simulink model "Robot_holonome_cinematique"  (R2023a)
settings: Solver=VariableStepAuto  StartTime=0.0  StopTime=1000  RelTol=1e-3
libraries: slpidlib x4
settings Model: Creator=Matth_desm  LastModifiedBy=maxen
settings OptimizationCC: ReuseModelBlockBuffer=off

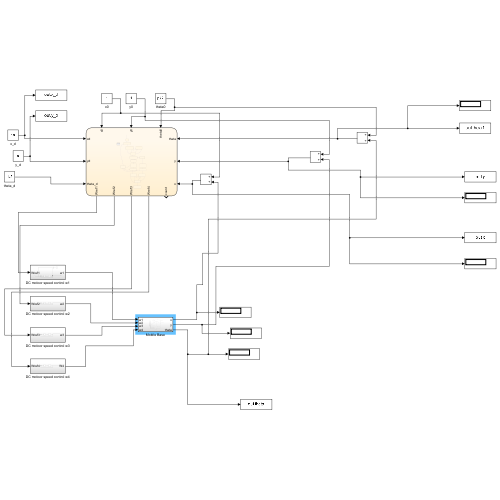
[thumbnail: Simulink's stored preview of the top-level diagram]
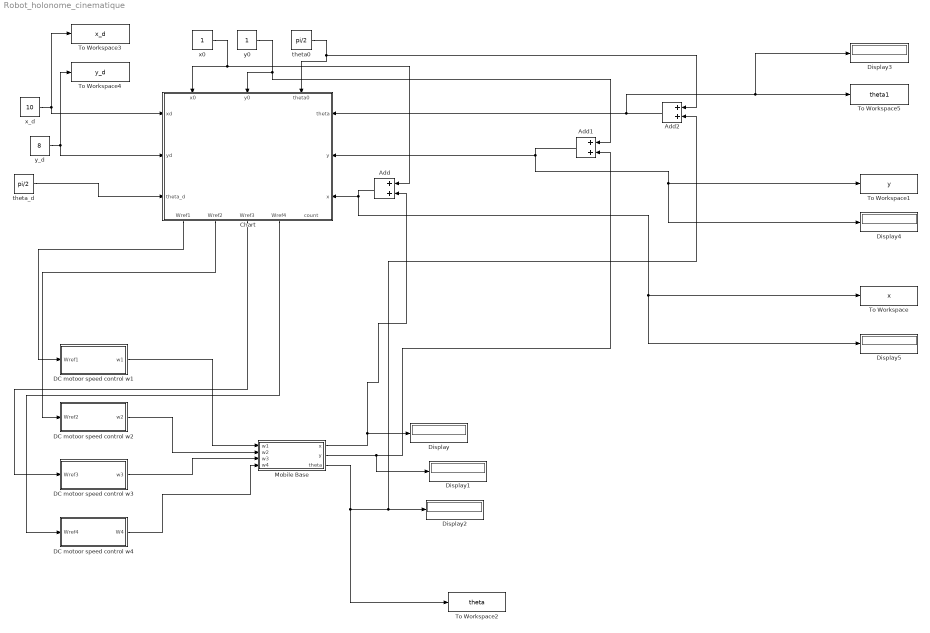
== system Robot_holonome_cinematique ==
  Add : Sum
  Add1 : Sum
  Add2 : Sum
  Chart : Stateflow chart  TreatAsAtomicUnit=on
      settings: PortSchema="{\"entries\":[{\"content\":{\"sides\":[{\"content\":{\"connectorIds\":[\"In5\",\"In6\",\"In3\"]},\"type\":\"ConnectorPlacement.EquallySpacedRectSide\",\"uuid\":\"9417ab48-c329-4538-ba36-cc7ccac6749b\"},{\"content\":{\"connectorIds\":[\"In7\",\"In8\",\"In9\"],\"side\":\"RIGHT\"},\"type\":\"ConnectorPlacement.EquallySpacedRectSide\",\"uuid\":\"8b0a8ded-c0e2-4ff2-a6eb-d9a6348e4391\"},{\"content\":{\"connectorIds\":[\"In1\",\"In2\",\"In4\"],\"side\":\"TOP\"},\"type\":\"ConnectorPlacement.EquallySpacedRectSide\",\"uuid\":\"84ebfe46-ef81-4416-a451-5548631499de\"},{\"content\":{\"connectorIds\":[\"Out1\",\"Out2\",\"Out3\",\"Out4\",\"Out5\"],\"side\":\"BOTTOM\"},\"type\":\"ConnectorPlacement.EquallySpacedRectSide\",\"uuid\":\"1f624b61-eefa-4aff-88e0-d3df134729c6\"}]},\"type\":\"ConnectorPlacement.EquallySpacedConnector\",\"uuid\":\"6488da51-1d08-4ec7-a718-29c3efed2e7e\"}],\"packageUris\":[\"http://schema.mathworks.com/mf0/Connector/R2020b\"],\"version\":\"1.0\"}"
  DC motoor speed control w1 : Subsystem
  DC motoor speed control w2 : Subsystem
  DC motoor speed control w3 : Subsystem
  DC motoor speed control w4 : Subsystem
  Display{,1..5} (6 alike) : Display
  Mobile Base : Subsystem
  To Workspace : ToWorkspace  VariableName=x  SampleTime=-1
      settings: Save2DSignal=2-D array (concatenate along first dimension)
  To Workspace1 : ToWorkspace  VariableName=y  SampleTime=-1
      settings: Save2DSignal=2-D array (concatenate along first dimension)
  To Workspace2 : ToWorkspace  VariableName=theta  SampleTime=-1
      settings: Save2DSignal=2-D array (concatenate along first dimension)
  To Workspace3 : ToWorkspace  VariableName=x_d  SampleTime=-1
      settings: Save2DSignal=2-D array (concatenate along first dimension)
  To Workspace4 : ToWorkspace  VariableName=y_d  SampleTime=-1
      settings: Save2DSignal=2-D array (concatenate along first dimension)
  To Workspace5 : ToWorkspace  VariableName=theta1  SampleTime=-1
      settings: Save2DSignal=2-D array (concatenate along first dimension)
  theta0 : Constant  Value=pi/2
  theta_d : Constant  Value=pi/2
  x0 : Constant
  x_d : Constant  Value=10
  y0 : Constant
  y_d : Constant  Value=8
  wires:
  DC motoor speed control w2/1(w2) -> Mobile Base/2(w2)
  DC motoor speed control w4/1(W4) -> Mobile Base/4(w4)
  Mobile Base/2(y) -> Add1/2, Display1/1
  DC motoor speed control w1/1(w1) -> Mobile Base/1(w1)
  Mobile Base/3(theta) -> To Workspace2/1, Add2/2, Display2/1
  Mobile Base/1(x) -> Add/2, Display/1
  DC motoor speed control w3/1(w3) -> Mobile Base/3(w3)
  theta0/1 -> Add2/1, Chart/4(theta0)
  x_d/1 -> To Workspace3/1, Chart/5(xd)
  theta_d/1 -> Chart/3(theta_d)
  y0/1 -> Add1/1, Chart/2(y0)
  x0/1 -> Add/1, Chart/1(x0)
  y_d/1 -> Chart/6(yd), To Workspace4/1
  Chart/1(Wref1) -> DC motoor speed control w1/1(Wref1)
  Chart/2(Wref2) -> DC motoor speed control w2/1(Wref2)
  Chart/3(Wref3) -> DC motoor speed control w3/1(Wref3)
  Chart/4(Wref4) -> DC motoor speed control w4/1(Wref4)
  Add1/1 -> Display4/1, To Workspace1/1, Chart/8(y)
  Add/1 -> Display5/1, To Workspace/1, Chart/9(x)
  Add2/1 -> Display3/1, To Workspace5/1, Chart/7(theta)

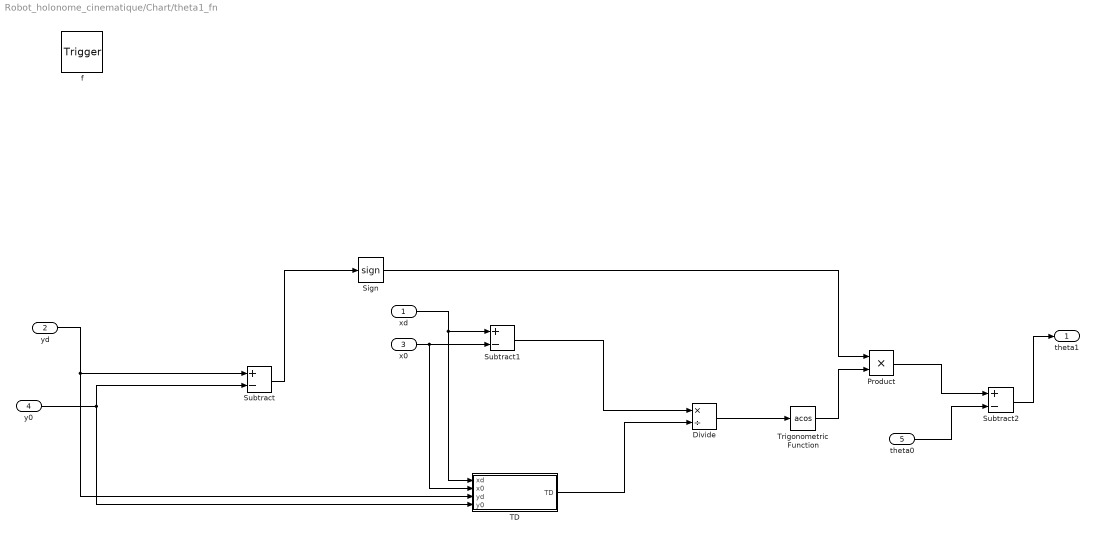
== system Robot_holonome_cinematique/Chart/theta1_fn ==
  xd : Inport  OutDataTypeStr=double  PortDimensions=1
  yd : Inport  Port=2  OutDataTypeStr=double  PortDimensions=1  LockScale=on
  x0 : Inport  Port=3  OutDataTypeStr=double  PortDimensions=1
  y0 : Inport  Port=4  OutDataTypeStr=double  PortDimensions=1
  theta0 : Inport  Port=5  OutDataTypeStr=double  PortDimensions=1
  f : TriggerPort  TriggerType=function-call  VariantControl=(inherit)
      settings: CopyFcn=Stateflow.SLINSF.SimulinkMan.removeBlockPreDeleteFcn  PreDeleteFcn=Stateflow.SLINSF.SimulinkMan.unsafePredeleteFcn
  Divide : Product  Inputs=*/
  Product : Product
  Sign : Signum
  Subtract : Sum  Inputs=+-
  Subtract1 : Sum  Inputs=+-
  Subtract2 : Sum  Inputs=+-
  TD : Subsystem
  Trigonometric Function : Trigonometry  Operator=acos
  theta1 : Outport  OutDataTypeStr=double
  wires:
  Trigonometric Function/1 -> Product/2
  TD/1(TD) -> Divide/2
  Sign/1 -> Product/1
  y0/1 -> TD/4(y0), Subtract/2
  Divide/1 -> Trigonometric Function/1
  Subtract1/1 -> Divide/1
  x0/1 -> TD/2(x0), Subtract1/2
  Subtract/1 -> Sign/1
  yd/1 -> TD/3(yd), Subtract/1
  xd/1 -> TD/1(xd), Subtract1/1
  Subtract2/1 -> theta1/1
  theta0/1 -> Subtract2/2
  Product/1 -> Subtract2/1

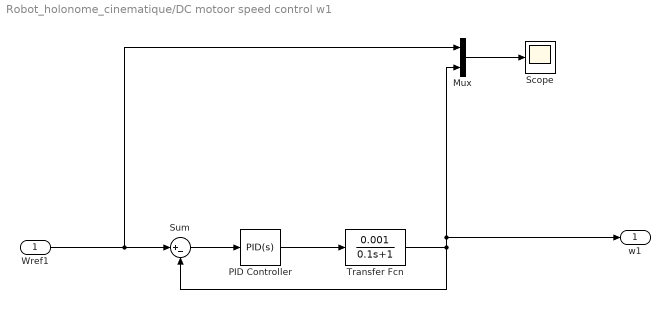
== system Robot_holonome_cinematique/DC motoor speed control w1 ==
  Wref1 : Inport
  Mux : Mux  Inputs=2
  PID Controller : slpidlib/PID Controller  Controller=PID  Form=Parallel  TimeDomain=Continuous-time  UseExternalTs=off  SampleTime=-1  IntegratorMethod=Forward Euler  FilterMethod=Forward Euler  ControllerParametersSource=internal  P=1337.5803137951  I=26735.5246643925  UseKiTs=off  D=-4.85758916096801  N=37.8094165182863  UseFilter=on  TunerSelectOption=Transfer Function Based (PID Tuner App)  InitialConditionSource=internal  InitialConditionForIntegrator=0  InitialConditionForFilter=0  DifferentiatorICPrevScaledInput=0  ExternalReset=none  TrackingMode=off  Kt=1  LimitOutput=off  SatLimitsSource=internal  UpperSaturationLimit=inf  LowerSaturationLimit=-inf  LinearizeAsGain=on  AntiWindupMode=none  Kb=1  LimitIntegrator=off  UpperIntegratorSaturationLimit=inf  LowerIntegratorSaturationLimit=-inf  POutMin=[]  POutMax=[]  IOutMin=[]  IOutMax=[]  DOutMin=[]  DOutMax=[]  NOutMin=[]  NOutMax=[]  SumOutMin=[]  SumOutMax=[]  SaturationOutMin=[]  SaturationOutMax=[]  PParamMin=[]  PParamMax=[]  IParamMin=[]  IParamMax=[]  DParamMin=[]  DParamMax=[]  NParamMin=[]  NParamMax=[]  KbParamMin=[]  KbParamMax=[]  KtParamMin=[]  KtParamMax=[]  KbOutMin=[]  KbOutMax=[]  KtOutMin=[]  KtOutMax=[]  IntegratorOutMin=[]  IntegratorOutMax=[]  FilterOutMin=[]  FilterOutMax=[]  SumI1OutMin=[]  SumI1OutMax=[]  SumI2OutMin=[]  SumI2OutMax=[]  SumI3OutMin=[]  SumI3OutMax=[]  SumI4OutMin=[]  SumI4OutMax=[]  SumDOutMin=[]  SumDOutMax=[]  DifferentiatorOutMin=[]  DifferentiatorOutMax=[]  FilterDiffOutCoefMin=[]  FilterDiffOutCoefMax=[]  ReciprocalOutMin=[]  ReciprocalOutMax=[]  SumDenOutMin=[]  SumDenOutMax=[]  SumNumOutMin=[]  SumNumOutMax=[]  DivideOutMin=[]  DivideOutMax=[]  UdiffTsProdOutMin=[]  UdiffTsProdOutMax=[]  NTsProdOutMin=[]  NTsProdOutMax=[]  UintegralTsProdOutMin=[]  UintegralTsProdOutMax=[]  UngainTsProdOutMin=[]  UngainTsProdOutMax=[]  ClampingZeroOutDataTypeStr=Inherit: Inherit via back propagation  ClampingZeroOutMin=[]  ClampingZeroOutMax=[]  FilterDenConstantOutDataTypeStr=Inherit: Inherit via back propagation  FilterDenConstantOutMin=[]  FilterDenConstantOutMax=[]  PCopyOutDataTypeStr=Inherit: Inherit via back propagation  PCopyOutMin=[]  PCopyOutMax=[]  NCopyOutDataTypeStr=Inherit: Inherit via back propagation  NCopyOutMin=[]  NCopyOutMax=[]  IntegratorContinuousStateAttributes=''  IntegratorStateMustResolveToSignalObject=off  IntegratorRTWStateStorageClass=Auto  FilterContinuousStateAttributes=''  FilterStateMustResolveToSignalObject=off  FilterRTWStateStorageClass=Auto  ParallelPVariant=InternalParameters  IdealPVariant=Disabled  IVariant=InternalParameters  DVariant=InternalParameters  IntegratorVariant=Continuous  SatVariant=Disabled  AWVariant=Passthrough  PCopyVariant=Disabled  TRVariant=Disabled  FdbkBlocksVariant=Forward  IdealPFdbkVariant=Disabled  SatFdbkVariant=Disabled  DerivativeFilterVariant=ContFilter  NVariant=InternalParameters  NCopyVariant=Disabled  FilterICVariant=InternalICsFilter  IntegratorICVariant=InternalICs  ExternalResetVariant=Disabled  TRSumVariant=Passthrough  SumFdbkVariant=Disabled  SumVariant=Sum_PID  TsampFilterVariant=InternalTs  TsampNgainVariant=Passthrough  TsampIntegralVariant=Disabled_SignalSpec  ExternalSaturationOutDataTypeStr=Inherit: Same as second input
  Scope : Scope
  Sum : Sum  Inputs=|+-
  Transfer Fcn : TransferFcn  Numerator=0.001  Denominator=[0.1 1]
  w1 : Outport
  wires:
  PID Controller/1 -> Transfer Fcn/1
  Transfer Fcn/1 -> Mux/2, w1/1, Sum/2
  Sum/1 -> PID Controller/1
  Wref1/1 -> Mux/1, Sum/1
  Mux/1 -> Scope/1

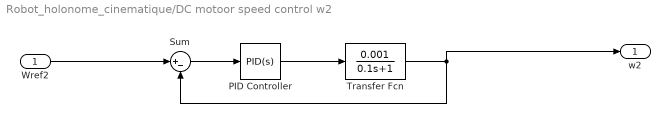
== system Robot_holonome_cinematique/DC motoor speed control w2 ==
  Wref2 : Inport
  PID Controller : slpidlib/PID Controller  Controller=PID  Form=Parallel  TimeDomain=Continuous-time  UseExternalTs=off  SampleTime=-1  IntegratorMethod=Forward Euler  FilterMethod=Forward Euler  ControllerParametersSource=internal  P=1337.5803137951  I=26735.5246643925  UseKiTs=off  D=-4.85758916096801  N=37.8094165182863  UseFilter=on  TunerSelectOption=Transfer Function Based (PID Tuner App)  InitialConditionSource=internal  InitialConditionForIntegrator=0  InitialConditionForFilter=0  DifferentiatorICPrevScaledInput=0  ExternalReset=none  TrackingMode=off  Kt=1  LimitOutput=off  SatLimitsSource=internal  UpperSaturationLimit=inf  LowerSaturationLimit=-inf  LinearizeAsGain=on  AntiWindupMode=none  Kb=1  LimitIntegrator=off  UpperIntegratorSaturationLimit=inf  LowerIntegratorSaturationLimit=-inf  POutMin=[]  POutMax=[]  IOutMin=[]  IOutMax=[]  DOutMin=[]  DOutMax=[]  NOutMin=[]  NOutMax=[]  SumOutMin=[]  SumOutMax=[]  SaturationOutMin=[]  SaturationOutMax=[]  PParamMin=[]  PParamMax=[]  IParamMin=[]  IParamMax=[]  DParamMin=[]  DParamMax=[]  NParamMin=[]  NParamMax=[]  KbParamMin=[]  KbParamMax=[]  KtParamMin=[]  KtParamMax=[]  KbOutMin=[]  KbOutMax=[]  KtOutMin=[]  KtOutMax=[]  IntegratorOutMin=[]  IntegratorOutMax=[]  FilterOutMin=[]  FilterOutMax=[]  SumI1OutMin=[]  SumI1OutMax=[]  SumI2OutMin=[]  SumI2OutMax=[]  SumI3OutMin=[]  SumI3OutMax=[]  SumI4OutMin=[]  SumI4OutMax=[]  SumDOutMin=[]  SumDOutMax=[]  DifferentiatorOutMin=[]  DifferentiatorOutMax=[]  FilterDiffOutCoefMin=[]  FilterDiffOutCoefMax=[]  ReciprocalOutMin=[]  ReciprocalOutMax=[]  SumDenOutMin=[]  SumDenOutMax=[]  SumNumOutMin=[]  SumNumOutMax=[]  DivideOutMin=[]  DivideOutMax=[]  UdiffTsProdOutMin=[]  UdiffTsProdOutMax=[]  NTsProdOutMin=[]  NTsProdOutMax=[]  UintegralTsProdOutMin=[]  UintegralTsProdOutMax=[]  UngainTsProdOutMin=[]  UngainTsProdOutMax=[]  ClampingZeroOutDataTypeStr=Inherit: Inherit via back propagation  ClampingZeroOutMin=[]  ClampingZeroOutMax=[]  FilterDenConstantOutDataTypeStr=Inherit: Inherit via back propagation  FilterDenConstantOutMin=[]  FilterDenConstantOutMax=[]  PCopyOutDataTypeStr=Inherit: Inherit via back propagation  PCopyOutMin=[]  PCopyOutMax=[]  NCopyOutDataTypeStr=Inherit: Inherit via back propagation  NCopyOutMin=[]  NCopyOutMax=[]  IntegratorContinuousStateAttributes=''  IntegratorStateMustResolveToSignalObject=off  IntegratorRTWStateStorageClass=Auto  FilterContinuousStateAttributes=''  FilterStateMustResolveToSignalObject=off  FilterRTWStateStorageClass=Auto  ParallelPVariant=InternalParameters  IdealPVariant=Disabled  IVariant=InternalParameters  DVariant=InternalParameters  IntegratorVariant=Continuous  SatVariant=Disabled  AWVariant=Passthrough  PCopyVariant=Disabled  TRVariant=Disabled  FdbkBlocksVariant=Forward  IdealPFdbkVariant=Disabled  SatFdbkVariant=Disabled  DerivativeFilterVariant=ContFilter  NVariant=InternalParameters  NCopyVariant=Disabled  FilterICVariant=InternalICsFilter  IntegratorICVariant=InternalICs  ExternalResetVariant=Disabled  TRSumVariant=Passthrough  SumFdbkVariant=Disabled  SumVariant=Sum_PID  TsampFilterVariant=InternalTs  TsampNgainVariant=Passthrough  TsampIntegralVariant=Disabled_SignalSpec  ExternalSaturationOutDataTypeStr=Inherit: Same as second input
  Sum : Sum  Inputs=|+-
  Transfer Fcn : TransferFcn  Numerator=0.001  Denominator=[0.1 1]
  w2 : Outport
  wires:
  PID Controller/1 -> Transfer Fcn/1
  Transfer Fcn/1 -> w2/1, Sum/2
  Sum/1 -> PID Controller/1
  Wref2/1 -> Sum/1

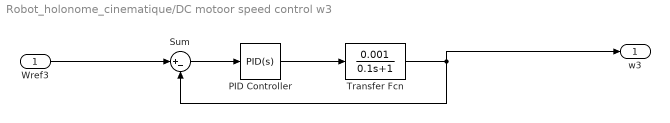
== system Robot_holonome_cinematique/DC motoor speed control w3 ==
  Wref3 : Inport
  PID Controller : slpidlib/PID Controller  Controller=PID  Form=Parallel  TimeDomain=Continuous-time  UseExternalTs=off  SampleTime=-1  IntegratorMethod=Forward Euler  FilterMethod=Forward Euler  ControllerParametersSource=internal  P=1337.5803137951  I=26735.5246643925  UseKiTs=off  D=-4.85758916096801  N=37.8094165182863  UseFilter=on  TunerSelectOption=Transfer Function Based (PID Tuner App)  InitialConditionSource=internal  InitialConditionForIntegrator=0  InitialConditionForFilter=0  DifferentiatorICPrevScaledInput=0  ExternalReset=none  TrackingMode=off  Kt=1  LimitOutput=off  SatLimitsSource=internal  UpperSaturationLimit=inf  LowerSaturationLimit=-inf  LinearizeAsGain=on  AntiWindupMode=none  Kb=1  LimitIntegrator=off  UpperIntegratorSaturationLimit=inf  LowerIntegratorSaturationLimit=-inf  POutMin=[]  POutMax=[]  IOutMin=[]  IOutMax=[]  DOutMin=[]  DOutMax=[]  NOutMin=[]  NOutMax=[]  SumOutMin=[]  SumOutMax=[]  SaturationOutMin=[]  SaturationOutMax=[]  PParamMin=[]  PParamMax=[]  IParamMin=[]  IParamMax=[]  DParamMin=[]  DParamMax=[]  NParamMin=[]  NParamMax=[]  KbParamMin=[]  KbParamMax=[]  KtParamMin=[]  KtParamMax=[]  KbOutMin=[]  KbOutMax=[]  KtOutMin=[]  KtOutMax=[]  IntegratorOutMin=[]  IntegratorOutMax=[]  FilterOutMin=[]  FilterOutMax=[]  SumI1OutMin=[]  SumI1OutMax=[]  SumI2OutMin=[]  SumI2OutMax=[]  SumI3OutMin=[]  SumI3OutMax=[]  SumI4OutMin=[]  SumI4OutMax=[]  SumDOutMin=[]  SumDOutMax=[]  DifferentiatorOutMin=[]  DifferentiatorOutMax=[]  FilterDiffOutCoefMin=[]  FilterDiffOutCoefMax=[]  ReciprocalOutMin=[]  ReciprocalOutMax=[]  SumDenOutMin=[]  SumDenOutMax=[]  SumNumOutMin=[]  SumNumOutMax=[]  DivideOutMin=[]  DivideOutMax=[]  UdiffTsProdOutMin=[]  UdiffTsProdOutMax=[]  NTsProdOutMin=[]  NTsProdOutMax=[]  UintegralTsProdOutMin=[]  UintegralTsProdOutMax=[]  UngainTsProdOutMin=[]  UngainTsProdOutMax=[]  ClampingZeroOutDataTypeStr=Inherit: Inherit via back propagation  ClampingZeroOutMin=[]  ClampingZeroOutMax=[]  FilterDenConstantOutDataTypeStr=Inherit: Inherit via back propagation  FilterDenConstantOutMin=[]  FilterDenConstantOutMax=[]  PCopyOutDataTypeStr=Inherit: Inherit via back propagation  PCopyOutMin=[]  PCopyOutMax=[]  NCopyOutDataTypeStr=Inherit: Inherit via back propagation  NCopyOutMin=[]  NCopyOutMax=[]  IntegratorContinuousStateAttributes=''  IntegratorStateMustResolveToSignalObject=off  IntegratorRTWStateStorageClass=Auto  FilterContinuousStateAttributes=''  FilterStateMustResolveToSignalObject=off  FilterRTWStateStorageClass=Auto  ParallelPVariant=InternalParameters  IdealPVariant=Disabled  IVariant=InternalParameters  DVariant=InternalParameters  IntegratorVariant=Continuous  SatVariant=Disabled  AWVariant=Passthrough  PCopyVariant=Disabled  TRVariant=Disabled  FdbkBlocksVariant=Forward  IdealPFdbkVariant=Disabled  SatFdbkVariant=Disabled  DerivativeFilterVariant=ContFilter  NVariant=InternalParameters  NCopyVariant=Disabled  FilterICVariant=InternalICsFilter  IntegratorICVariant=InternalICs  ExternalResetVariant=Disabled  TRSumVariant=Passthrough  SumFdbkVariant=Disabled  SumVariant=Sum_PID  TsampFilterVariant=InternalTs  TsampNgainVariant=Passthrough  TsampIntegralVariant=Disabled_SignalSpec  ExternalSaturationOutDataTypeStr=Inherit: Same as second input
  Sum : Sum  Inputs=|+-
  Transfer Fcn : TransferFcn  Numerator=0.001  Denominator=[0.1 1]
  w3 : Outport
  wires:
  PID Controller/1 -> Transfer Fcn/1
  Transfer Fcn/1 -> w3/1, Sum/2
  Sum/1 -> PID Controller/1
  Wref3/1 -> Sum/1

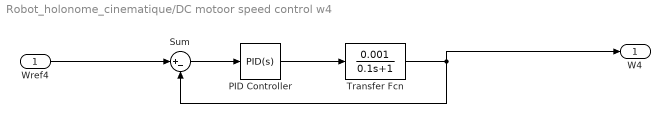
== system Robot_holonome_cinematique/DC motoor speed control w4 ==
  Wref4 : Inport
  PID Controller : slpidlib/PID Controller  Controller=PID  Form=Parallel  TimeDomain=Continuous-time  UseExternalTs=off  SampleTime=-1  IntegratorMethod=Forward Euler  FilterMethod=Forward Euler  ControllerParametersSource=internal  P=1337.5803137951  I=26735.5246643925  UseKiTs=off  D=-4.85758916096801  N=37.8094165182863  UseFilter=on  TunerSelectOption=Transfer Function Based (PID Tuner App)  InitialConditionSource=internal  InitialConditionForIntegrator=0  InitialConditionForFilter=0  DifferentiatorICPrevScaledInput=0  ExternalReset=none  TrackingMode=off  Kt=1  LimitOutput=off  SatLimitsSource=internal  UpperSaturationLimit=inf  LowerSaturationLimit=-inf  LinearizeAsGain=on  AntiWindupMode=none  Kb=1  LimitIntegrator=off  UpperIntegratorSaturationLimit=inf  LowerIntegratorSaturationLimit=-inf  POutMin=[]  POutMax=[]  IOutMin=[]  IOutMax=[]  DOutMin=[]  DOutMax=[]  NOutMin=[]  NOutMax=[]  SumOutMin=[]  SumOutMax=[]  SaturationOutMin=[]  SaturationOutMax=[]  PParamMin=[]  PParamMax=[]  IParamMin=[]  IParamMax=[]  DParamMin=[]  DParamMax=[]  NParamMin=[]  NParamMax=[]  KbParamMin=[]  KbParamMax=[]  KtParamMin=[]  KtParamMax=[]  KbOutMin=[]  KbOutMax=[]  KtOutMin=[]  KtOutMax=[]  IntegratorOutMin=[]  IntegratorOutMax=[]  FilterOutMin=[]  FilterOutMax=[]  SumI1OutMin=[]  SumI1OutMax=[]  SumI2OutMin=[]  SumI2OutMax=[]  SumI3OutMin=[]  SumI3OutMax=[]  SumI4OutMin=[]  SumI4OutMax=[]  SumDOutMin=[]  SumDOutMax=[]  DifferentiatorOutMin=[]  DifferentiatorOutMax=[]  FilterDiffOutCoefMin=[]  FilterDiffOutCoefMax=[]  ReciprocalOutMin=[]  ReciprocalOutMax=[]  SumDenOutMin=[]  SumDenOutMax=[]  SumNumOutMin=[]  SumNumOutMax=[]  DivideOutMin=[]  DivideOutMax=[]  UdiffTsProdOutMin=[]  UdiffTsProdOutMax=[]  NTsProdOutMin=[]  NTsProdOutMax=[]  UintegralTsProdOutMin=[]  UintegralTsProdOutMax=[]  UngainTsProdOutMin=[]  UngainTsProdOutMax=[]  ClampingZeroOutDataTypeStr=Inherit: Inherit via back propagation  ClampingZeroOutMin=[]  ClampingZeroOutMax=[]  FilterDenConstantOutDataTypeStr=Inherit: Inherit via back propagation  FilterDenConstantOutMin=[]  FilterDenConstantOutMax=[]  PCopyOutDataTypeStr=Inherit: Inherit via back propagation  PCopyOutMin=[]  PCopyOutMax=[]  NCopyOutDataTypeStr=Inherit: Inherit via back propagation  NCopyOutMin=[]  NCopyOutMax=[]  IntegratorContinuousStateAttributes=''  IntegratorStateMustResolveToSignalObject=off  IntegratorRTWStateStorageClass=Auto  FilterContinuousStateAttributes=''  FilterStateMustResolveToSignalObject=off  FilterRTWStateStorageClass=Auto  ParallelPVariant=InternalParameters  IdealPVariant=Disabled  IVariant=InternalParameters  DVariant=InternalParameters  IntegratorVariant=Continuous  SatVariant=Disabled  AWVariant=Passthrough  PCopyVariant=Disabled  TRVariant=Disabled  FdbkBlocksVariant=Forward  IdealPFdbkVariant=Disabled  SatFdbkVariant=Disabled  DerivativeFilterVariant=ContFilter  NVariant=InternalParameters  NCopyVariant=Disabled  FilterICVariant=InternalICsFilter  IntegratorICVariant=InternalICs  ExternalResetVariant=Disabled  TRSumVariant=Passthrough  SumFdbkVariant=Disabled  SumVariant=Sum_PID  TsampFilterVariant=InternalTs  TsampNgainVariant=Passthrough  TsampIntegralVariant=Disabled_SignalSpec  ExternalSaturationOutDataTypeStr=Inherit: Same as second input
  Sum : Sum  Inputs=|+-
  Transfer Fcn : TransferFcn  Numerator=0.001  Denominator=[0.1 1]
  W4 : Outport
  wires:
  PID Controller/1 -> Transfer Fcn/1
  Transfer Fcn/1 -> W4/1, Sum/2
  Sum/1 -> PID Controller/1
  Wref4/1 -> Sum/1

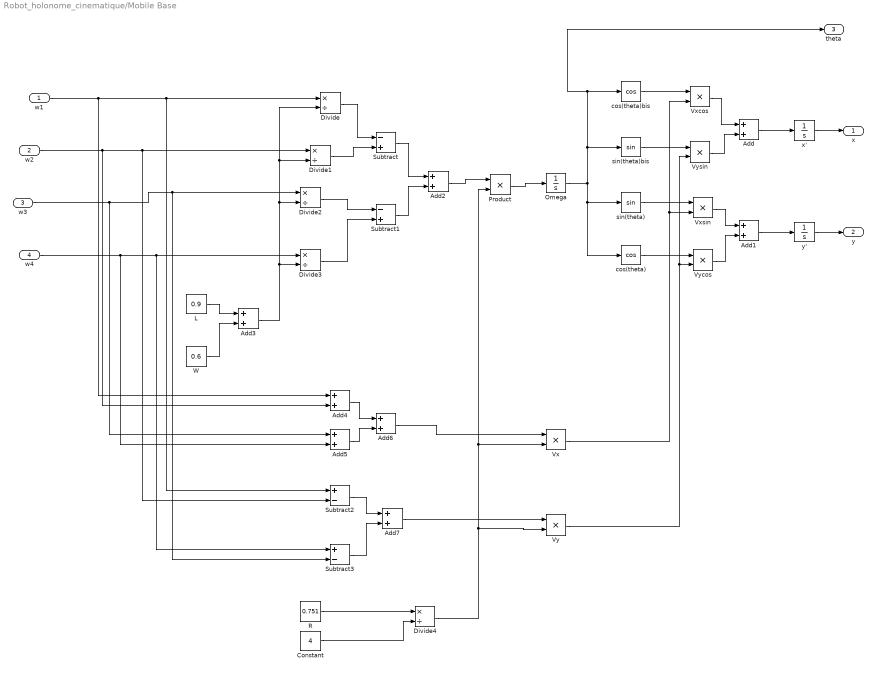
== system Robot_holonome_cinematique/Mobile Base ==
  w1 : Inport
  w2 : Inport  Port=2
  w3 : Inport  Port=3
  w4 : Inport  Port=4
  " cos(theta)" : Trigonometry  Operator=cos
  Add{,1..7} (8 alike) : Sum
  Constant : Constant  Value=4
  Divide{,1..4} (5 alike) : Product  Inputs=*/
  L : Constant  Value=0.9
  Omega : Integrator
  Product : Product
  R : Constant  Value=0.751
  Subtract : Sum  Inputs=-+
  Subtract1 : Sum  Inputs=-+
  Subtract2 : Sum  Inputs=+-
  Subtract3 : Sum  Inputs=+-
  Vx : Product
  Vxcos : Product
  Vxsin : Product
  Vy : Product
  Vycos : Product
  Vysin : Product
  W : Constant  Value=0.6
  cos(theta)bis : Trigonometry  Operator=cos
  sin(theta) : Trigonometry
  sin(theta)bis : Trigonometry
  x' : Integrator
  y' : Integrator
  x : Outport
  y : Outport  Port=2
  theta : Outport  Port=3
  wires:
  x'/1 -> x/1
  y'/1 -> y/1
  " cos(theta)"/1 -> Vycos/1
  sin(theta)/1 -> Vxsin/1
  sin(theta)bis/1 -> Vysin/1
  cos(theta)bis/1 -> Vxcos/1
  Add1/1 -> y'/1
  Add/1 -> x'/1
  Vysin/1 -> Add/2
  Vxcos/1 -> Add/1
  Vxsin/1 -> Add1/1
  Vycos/1 -> Add1/2
  Omega/1 -> " cos(theta)"/1, sin(theta)/1, sin(theta)bis/1, theta/1, cos(theta)bis/1
  Subtract1/1 -> Add2/2
  Subtract/1 -> Add2/1
  w3/1 -> Add5/1, Subtract3/2, Divide2/1
  w4/1 -> Add5/2, Subtract3/1, Divide3/1
  w2/1 -> Add4/2, Subtract2/2, Divide1/1
  w1/1 -> Divide/1, Subtract2/1, Add4/1
  Divide/1 -> Subtract/1
  Divide1/1 -> Subtract/2
  Divide2/1 -> Subtract1/1
  Divide3/1 -> Subtract1/2
  L/1 -> Add3/1
  W/1 -> Add3/2
  Add3/1 -> Divide3/2, Divide2/2, Divide1/2, Divide/2
  Add5/1 -> Add6/2
  Add4/1 -> Add6/1
  Product/1 -> Omega/1
  Add2/1 -> Product/1
  R/1 -> Divide4/1
  Constant/1 -> Divide4/2
  Divide4/1 -> Vy/2, Vx/2, Product/2
  Add6/1 -> Vx/1
  Subtract2/1 -> Add7/1
  Subtract3/1 -> Add7/2
  Add7/1 -> Vy/1
  Vx/1 -> Vxsin/2, Vxcos/2
  Vy/1 -> Vysin/2, Vycos/2

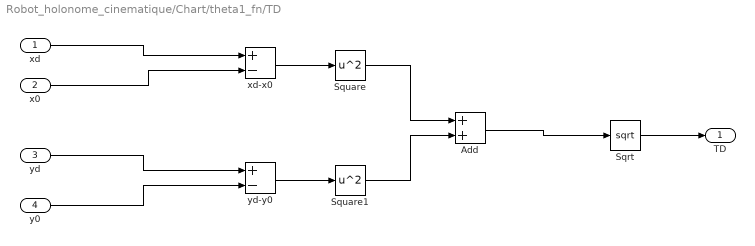
== system Robot_holonome_cinematique/Chart/theta1_fn/TD ==
  xd : Inport
  x0 : Inport  Port=2
  yd : Inport  Port=3
  y0 : Inport  Port=4
  Add : Sum
  Sqrt : Sqrt
  Square : Math  Operator=square
  Square1 : Math  Operator=square
  xd-x0 : Sum  Inputs=+-
  yd-y0 : Sum  Inputs=+-
  TD : Outport
  wires:
  xd/1 -> xd-x0/1
  x0/1 -> xd-x0/2
  yd/1 -> yd-y0/1
  y0/1 -> yd-y0/2
  yd-y0/1 -> Square1/1
  xd-x0/1 -> Square/1
  Square/1 -> Add/1
  Square1/1 -> Add/2
  Add/1 -> Sqrt/1
  Sqrt/1 -> TD/1

== stateflow chart Robot_holonome_cinematique/Chart ==
  state Debut
    entry:
    xdep=x0
    ydep=x0
    theta_dep=theta0
    count=1;
  state preparation
    entry:
    theta1=theta1_fn(xd,yd,xdep,ydep,theta_dep)
    theta1+theta0
  state theta1 = theta1_fn(xd,yd,x0,y0,theta0) [function]
  state Tourner
    entry:
    Wref1=-0.05;
    Wref2=0.05;
    Wref3=-0.05;
    Wref4=0.05;
    theta
  state Tourner_sens_inverse
    entry:
    Wref1=0.05;
    Wref2=-0.05;
    Wref3=0.05;
    Wref4=-0.05;
    theta
  state test_angle
    Wref1
  state Ligne_droite
    entry:
    Wref1=0.05;
    Wref2=0.05;
    Wref3=0.05;
    Wref4=0.05;
  state test_grandeur_x_y1
  state test_grandeur_x_y
  state Test_en_x
    entry:
    x
    y
    Wref1=0;
    Wref2=0;
    Wref3=0;
    Wref4=0;
  state Test_en_y
    entry:
    x
    y
    Wref1=0;
    Wref2=0;
    Wref3=0;
    Wref4=0;
  state Correction
    xdep=x;
    ydep=y
    theta_dep=theta
  state Test_y
    theta1
  state Test_x
    theta1
  state Tourner_fin
    entry:
    Wref1=-0.05;
    Wref2=0.05;
    Wref3=-0.05;
    Wref4=0.05;
    theta
  state Tourner_fin1
    entry:
    Wref1=0.05;
    Wref2=-0.05;
    Wref3=0.05;
    Wref4=-0.05;
    theta
  state test_angle_fin
    theta_d
  state Fin
    entry:
    Wref1=0;
    Wref2=0;
    Wref3=0;
    Wref4=0;
    x
    y
    theta
  (default) -> Debut
  Debut -> preparation
  Correction -> preparation
  preparation -> Tourner
  Tourner_sens_inverse -> Tourner_sens_inverse [order 2]
  Tourner -> Tourner [order 2]
  Tourner_sens_inverse -> test_angle [order 1] : [theta<=(theta1+theta0)+0.001]
  test_angle -> Tourner_sens_inverse [order 1] : [theta>(theta1+theta0)+0.001]
  test_angle -> Tourner [order 2] : [theta<(theta1+theta0)-0.001]
  Tourner -> test_angle [order 1] : [theta>=(theta1+theta0)-0.001]
  test_angle -> Ligne_droite [order 3]
  Ligne_droite -> test_grandeur_x_y1 [order 2]
  test_grandeur_x_y1 -> Test_en_y : [abs(y)>=abs(yd-0.05)]
  Ligne_droite -> test_grandeur_x_y [order 1] : [abs(x)>=abs(y)]
  test_grandeur_x_y -> Test_en_x : [abs(x)>=abs(xd-0.05)]
  Test_en_x -> Correction [order 2]
  Test_en_x -> Test_y [order 1] : [abs(yd-1)<abs(y)]
  Test_en_y -> Test_x : [abs(xd-1)<abs(x)]
  Test_x -> Correction [order 1] : [abs(x)>abs(xd+1)]
  Test_y -> Correction [order 1] : [y>yd+1]
  Test_y -> Tourner_fin [order 2]
  Test_x -> Tourner_fin1 [order 2]
  Tourner_fin -> Tourner_fin [order 2]
  Tourner_fin1 -> Tourner_fin1 [order 2]
  test_angle_fin -> Tourner_fin [order 2] : [theta<=theta_d-0.01]
  Tourner_fin -> test_angle_fin [order 1] : [theta>=theta_d-0.001]
  Tourner_fin1 -> test_angle_fin [order 1] : [theta<=theta_d+0.001]
  test_angle_fin -> Tourner_fin1 [order 1] : [theta>=theta_d+0.001]
  test_angle_fin -> Fin [order 3]
  data: xd function_input double size=1; yd function_input double size=1; x0 function_input double size=1; y0 function_input double size=1; theta0 function_input double size=1; theta1 function_output double; x0 input; y0 input; theta_d input; theta0 input; xd input; yd input; theta input; y input; Wref1 output; Wref2 output; x input; theta1 local; xdep local; ydep local; theta_dep local; Wref3 output; Wref4 output; count output
